simulink model "rover_rocker_bogie"  (R2021a)
settings: Solver=ode23t  StartTime=0.0  StopTime=1e-2  RelTol=1e-3
values from neighbouring files (symbols this model uses):
  s = tf('s')    [Apollo_LM_design_discrete_observer.m]    (also in elastic_shaft_rlocus.m; harmonic_osc_rlocus.m)
undefined symbols (not defined in the file or in its folder): X, Y, Z
libraries: sm_lib x51, nesl_utility x11
(part 1 of 2)
settings Model: Creator=kjartan  LastModifiedBy=kjartan

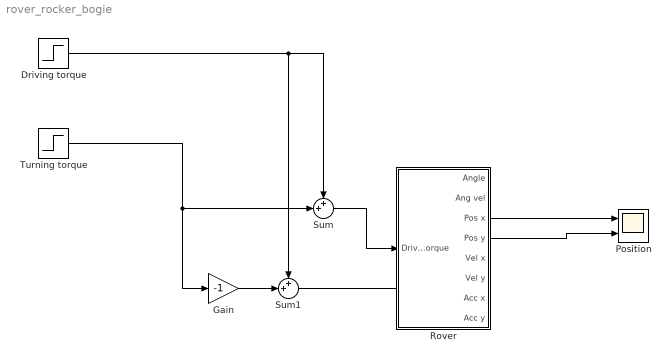
== system rover_rocker_bogie ==
  Driving torque : Step  Time=0  After=100  SampleTime=0
  Gain : Gain  Gain=-1
  Position : Scope  NumInputPorts=2
  Rover : Subsystem
  Sum : Sum  Inputs=++|
  Sum1 : Sum  Inputs=++|
  Turning torque : Step  After=30  SampleTime=0
  wires:
  Turning torque/1 -> Sum/2, Gain/1
  Sum/1 -> Rover/1(Driving torque)
  Driving torque/1 -> Sum1/1, Sum/1
  Gain/1 -> Sum1/2
  Sum1/1 -> ?
  Rover/3(Pos x) -> Position/1
  Rover/4(Pos y) -> Position/2
